simulink model "Q3_Lyap"  (R2021b)
settings: Solver=VariableStepAuto  StartTime=0.0  StopTime=2000  MaxStep=0.01  MinStep=0.001  RelTol=1e-3
model workspace (MAT data in the model file):
  a = -1
settings Model: PacingRate=1000  Creator=MAHDI  LastModifiedBy=YSNsec

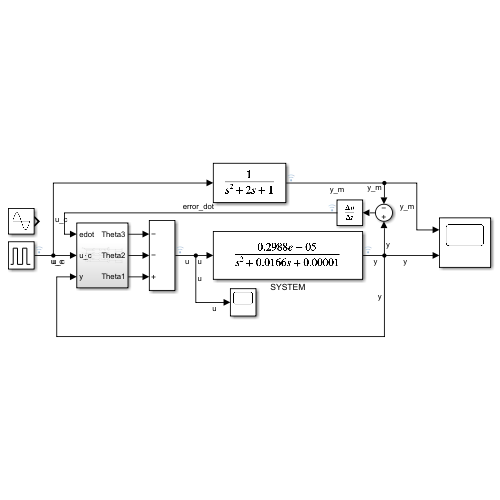
[thumbnail: Simulink's stored preview of the top-level diagram]
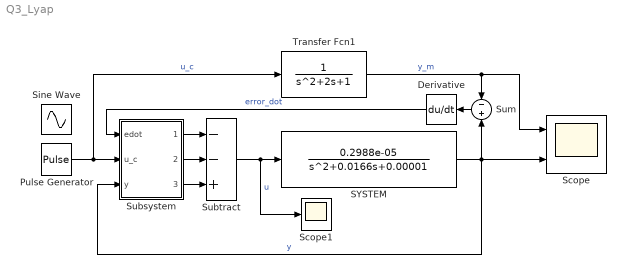
== system Q3_Lyap ==
  Derivative : Derivative
  Pulse Generator : DiscretePulseGenerator  PulseType=Time based  Amplitude=50  Period=200  PulseWidth=50  VectorParams1D=off
  SYSTEM : TransferFcn  Numerator=0.2988e-05  Denominator=[1 0.0166 0.00001]
  Scope : Scope  NumInputPorts=2
  Scope1 : Scope
  Sine Wave : Sin  Amplitude=10  Frequency=0.01  SampleTime=0
  Subsystem : Subsystem
  Subtract : Sum  Inputs=--+
  Sum : Sum  Inputs=-|+
  Transfer Fcn1 : TransferFcn
  wires:
  Pulse Generator/1 -> Transfer Fcn1/1, Subsystem/2(u_c)  "u_c"
  Subtract/1 -> SYSTEM/1, Scope1/1  "u"
  Transfer Fcn1/1 -> Scope/1, Sum/1  "y_m"
  SYSTEM/1 -> Scope/2, Subsystem/3(y), Sum/2  "y"
  Sum/1 -> Derivative/1
  Subsystem/1(Theta3) -> Subtract/1
  Subsystem/2(Theta2) -> Subtract/2
  Subsystem/3(Theta1) -> Subtract/3
  Derivative/1 -> Subsystem/1(edot)  "error_dot"

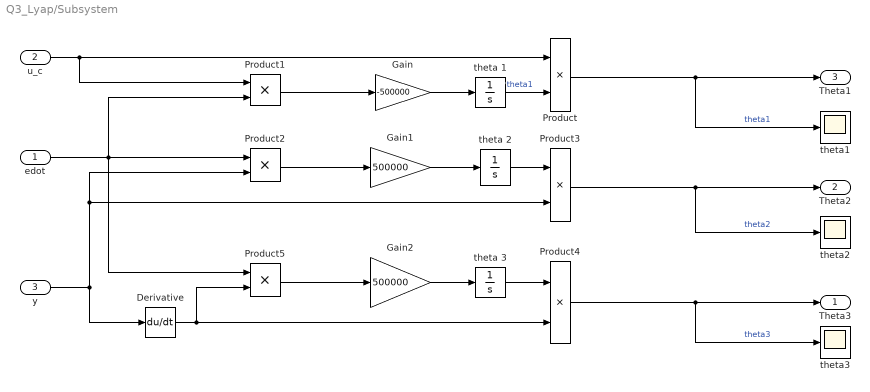
== system Q3_Lyap/Subsystem ==
  edot : Inport
  u_c : Inport  Port=2
  y : Inport  Port=3
  Derivative : Derivative
  Gain : Gain  Gain=-500000
  Gain1 : Gain  Gain=500000
  Gain2 : Gain  Gain=500000
  Product{,1..5} (6 alike) : Product
  theta 1 : Integrator
  theta 2 : Integrator
  theta 3 : Integrator
  theta1 : Scope
  theta2 : Scope
  theta3 : Scope
  Theta3 : Outport
  Theta2 : Outport  Port=2
  Theta1 : Outport  Port=3
  wires:
  Product3/1 -> theta2/1, Theta2/1  "theta2"
  y/1 -> Product2/2, Product3/2, Derivative/1
  Derivative/1 -> Product5/2, Product4/2
  Product5/1 -> Gain2/1
  theta 1/1 -> Product/2  "theta1"
  Gain2/1 -> theta 3/1
  edot/1 -> Product1/2, Product5/1, Product2/1
  Gain1/1 -> theta 2/1
  Product1/1 -> Gain/1
  Product/1 -> Theta1/1, theta1/1  "theta1"
  theta 3/1 -> Product4/1
  theta 2/1 -> Product3/1
  Product4/1 -> theta3/1, Theta3/1  "theta3"
  Gain/1 -> theta 1/1
  Product2/1 -> Gain1/1
  u_c/1 -> Product1/1, Product/1
